simulink model "p6"  (R2021b)
settings: Solver=VariableStepAuto  StartTime=0.0  StopTime=10.0  RelTol=1e-3
values from neighbouring files (symbols this model uses):
  A = [0 -0.378002311941 0 18.900115597 1 0 0 0 0 7.01473716863 0 -0.379715574203 ... (16 elements, 4x4)]    [Parameters.mat]
  B = [0 -0.0699290719413 0 3.49645359707]    [Parameters.mat]
  cx = [1 0 0 0]    [Parameters.mat]
  k_slow = [20.7523551145 9.40402411533 21.9918477145 2.35791844149]    [Parameters.mat]
  p_s = 15.3468449104    [Parameters.mat]
undefined symbols (not defined in the file or in its folder): CTinv, F, L_lyapanov, TB
settings Model: Creator=mahya  LastModifiedBy=mahya

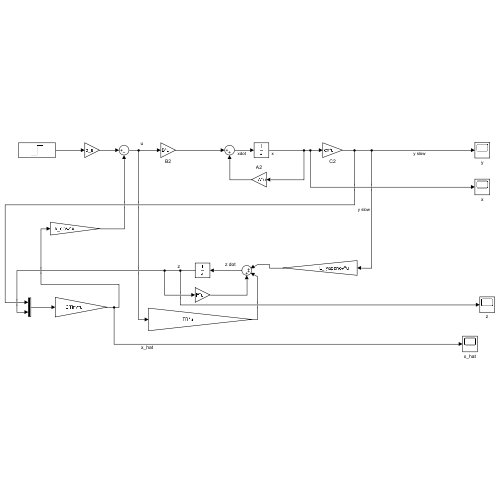
[thumbnail: Simulink's stored preview of the top-level diagram]
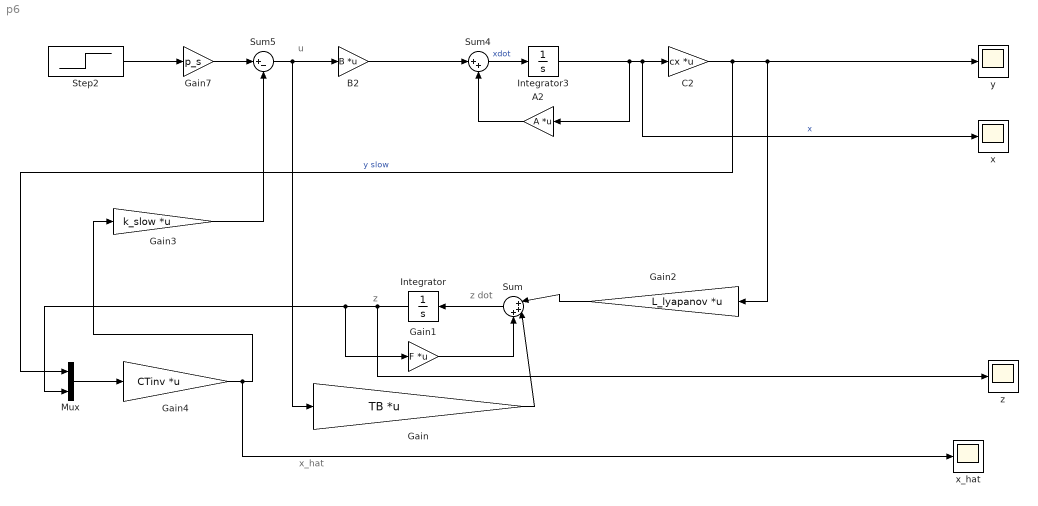
== system p6 ==
  note: x_hat
  note: u
  note: z
  note: z dot
  A2 : Gain  Gain=A  Multiplication=Matrix(K*u)
  B2 : Gain  Gain=B  Multiplication=Matrix(K*u)
  C2 : Gain  Gain=cx  Multiplication=Matrix(K*u)
  Gain : Gain  Gain=TB  Multiplication=Matrix(K*u)
  Gain1 : Gain  Gain=F  Multiplication=Matrix(K*u)
  Gain2 : Gain  Gain=L_lyapanov  Multiplication=Matrix(K*u)
  Gain3 : Gain  Gain=k_slow  Multiplication=Matrix(K*u)
  Gain4 : Gain  Gain=CTinv  Multiplication=Matrix(K*u)
  Gain7 : Gain  Gain=p_s
  Integrator : Integrator
  Integrator3 : Integrator  InitialCondition=[0 0 0 0]
  Mux : Mux  Inputs=2
  Step2 : Step  Time=0  SampleTime=0
  Sum : Sum  Inputs=|+++
  Sum4 : Sum  Inputs=|++
  Sum5 : Sum  Inputs=|+-
  x : Scope
  x_hat : Scope
  y : Scope
  z : Scope
  wires:
  B2/1 -> Sum4/1
  A2/1 -> Sum4/2
  Integrator3/1 -> A2/1, x/1, C2/1  "x"
  Step2/1 -> Gain7/1
  Sum4/1 -> Integrator3/1  "xdot"
  C2/1 -> Mux/1, Gain2/1, y/1  "y slow"
  Gain2/1 -> Sum/1
  Integrator/1 -> z/1, Mux/2, Gain1/1
  Gain1/1 -> Sum/3
  Gain/1 -> Sum/2
  Sum/1 -> Integrator/1
  Gain7/1 -> Sum5/1
  Sum5/1 -> Gain/1, B2/1
  Gain3/1 -> Sum5/2
  Mux/1 -> Gain4/1
  Gain4/1 -> x_hat/1, Gain3/1
